simulink model "SistemaP2"  (R2024b)
settings: Solver=ode15s  StartTime=0.0  StopTime=30  RelTol=1e-3
libraries: slpidlib x1
settings Model: LastModifiedBy=DELL
settings DataIOCC: ReturnWorkspaceOutputs=off  TimeSaveName=t
settings DebuggingCC: AlgebraicLoopMsg=none  ArtificialAlgebraicLoopMsg=none  MaxConsecutiveZCsMsg=none  OperatingPointInterfaceChecksumMismatchMsg=none

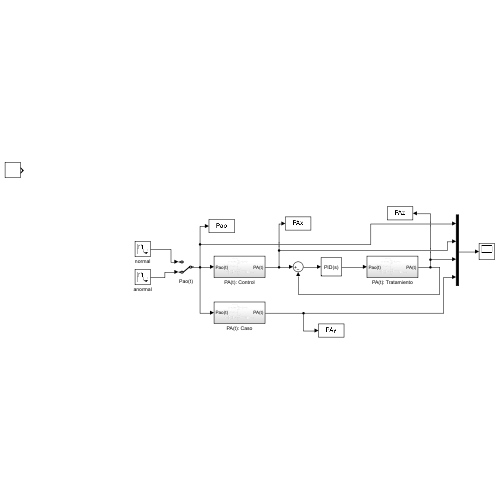
[thumbnail: Simulink's stored preview of the top-level diagram]
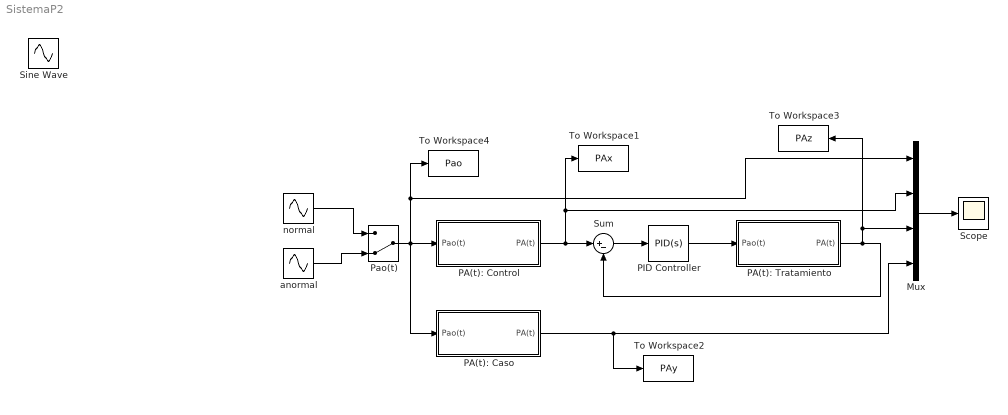
== system SistemaP2 ==
  Mux : Mux
  PA(t): Caso : Subsystem
  PA(t): Control : Subsystem
  PA(t): Tratamiento : Subsystem
  PID Controller : slpidlib/PID Controller  Controller=PID  Form=Parallel  TimeDomain=Continuous-time  UseExternalTs=off  SampleTime=-1  IntegratorMethod=Forward Euler  FilterMethod=Forward Euler  ControllerParametersSource=internal  P=151.384729406451  I=3438.58437249698  UseKiTs=off  D=0.496015778434629  UseExternalDerivativeSource=off  N=288.831749377284  UseFilter=on  TunerSelectOption=Transfer Function Based (PID Tuner App)  InitialConditionSource=internal  InitialConditionForIntegrator=0  InitialConditionForFilter=0  DifferentiatorICPrevScaledInput=0  ExternalReset=none  TrackingMode=off  Kt=1  LimitOutput=off  SatLimitsSource=internal  UpperSaturationLimit=inf  LowerSaturationLimit=-inf  LinearizeAsGain=on  AntiWindupMode=none  Kb=1  LimitIntegrator=off  UpperIntegratorSaturationLimit=inf  LowerIntegratorSaturationLimit=-inf  POutMin=[]  POutMax=[]  IOutMin=[]  IOutMax=[]  DOutMin=[]  DOutMax=[]  NOutMin=[]  NOutMax=[]  SumOutMin=[]  SumOutMax=[]  SaturationOutMin=[]  SaturationOutMax=[]  PParamMin=[]  PParamMax=[]  IParamMin=[]  IParamMax=[]  DParamMin=[]  DParamMax=[]  NParamMin=[]  NParamMax=[]  KbParamMin=[]  KbParamMax=[]  KtParamMin=[]  KtParamMax=[]  KbOutMin=[]  KbOutMax=[]  KtOutMin=[]  KtOutMax=[]  IntegratorOutMin=[]  IntegratorOutMax=[]  FilterOutMin=[]  FilterOutMax=[]  SumI1OutMin=[]  SumI1OutMax=[]  SumI2OutMin=[]  SumI2OutMax=[]  SumI3OutMin=[]  SumI3OutMax=[]  SumI4OutMin=[]  SumI4OutMax=[]  SumDOutMin=[]  SumDOutMax=[]  DifferentiatorOutMin=[]  DifferentiatorOutMax=[]  FilterDiffOutCoefMin=[]  FilterDiffOutCoefMax=[]  ReciprocalOutMin=[]  ReciprocalOutMax=[]  SumDenOutMin=[]  SumDenOutMax=[]  SumNumOutMin=[]  SumNumOutMax=[]  DivideOutMin=[]  DivideOutMax=[]  UdiffTsProdOutMin=[]  UdiffTsProdOutMax=[]  NTsProdOutMin=[]  NTsProdOutMax=[]  UintegralTsProdOutMin=[]  UintegralTsProdOutMax=[]  UngainTsProdOutMin=[]  UngainTsProdOutMax=[]  ClampingZeroOutDataTypeStr=Inherit: Inherit via back propagation  ClampingZeroOutMin=[]  ClampingZeroOutMax=[]  FilterDenConstantOutDataTypeStr=Inherit: Inherit via back propagation  FilterDenConstantOutMin=[]  FilterDenConstantOutMax=[]  PCopyOutDataTypeStr=Inherit: Inherit via back propagation  PCopyOutMin=[]  PCopyOutMax=[]  NCopyOutDataTypeStr=Inherit: Inherit via back propagation  NCopyOutMin=[]  NCopyOutMax=[]  IntegratorContinuousStateAttributes=''  IntegratorStateMustResolveToSignalObject=off  IntegratorRTWStateStorageClass=Auto  FilterContinuousStateAttributes=''  FilterStateMustResolveToSignalObject=off  FilterRTWStateStorageClass=Auto  ParallelPVariant=InternalParameters  IdealPVariant=Disabled  IVariant=InternalParameters  DVariant=InternalParameters  IntegratorVariant=Continuous  SatVariant=Disabled  AWVariant=Passthrough  PCopyVariant=Disabled  TRVariant=Disabled  FdbkBlocksVariant=Forward  IdealPFdbkVariant=Disabled  SatFdbkVariant=Disabled  DerivativeFilterVariant=ContFilter  NVariant=InternalParameters  NCopyVariant=Disabled  FilterICVariant=InternalICsFilter  IntegratorICVariant=InternalICs  ExternalResetVariant=Disabled  TRSumVariant=Passthrough  SumFdbkVariant=Disabled  SumVariant=Sum_PID  TsampFilterVariant=InternalTs  TsampNgainVariant=Passthrough  TsampIntegralVariant=Disabled_SignalSpec  ExternalSaturationOutDataTypeStr=Inherit: Same as second input  DerivativeSourceVariant=ErrorSignal  PreIntVariant=InternalPreInt
  Pao(t) : ManualSwitch  CurrentSetting=0
  Scope : Scope
  Sine Wave : Sin  Frequency=1.5708  SampleTime=0.001
  Sum : Sum  Inputs=|+-
  To Workspace1 : ToWorkspace  VariableName=PAx  SampleTime=-1
      settings: Save2DSignal=2-D array (concatenate along first dimension)
  To Workspace2 : ToWorkspace  VariableName=PAy  SampleTime=-1
      settings: Save2DSignal=2-D array (concatenate along first dimension)
  To Workspace3 : ToWorkspace  VariableName=PAz  SampleTime=-1
      settings: Save2DSignal=2-D array (concatenate along first dimension)
  To Workspace4 : ToWorkspace  VariableName=Pao  SampleTime=-1
      settings: Save2DSignal=2-D array (concatenate along first dimension)
  anormal : Sin  Amplitude=1.7  Frequency=pi  SampleTime=0.001
  normal : Sin  Amplitude=2.7  Frequency=pi/2  SampleTime=0.001
  wires:
  PA(t): Control/1(PA(t)) -> To Workspace1/1, Mux/2, Sum/1
  Sum/1 -> PID Controller/1
  Mux/1 -> Scope/1
  PA(t): Caso/1(PA(t)) -> To Workspace2/1, Mux/4
  PA(t): Tratamiento/1(PA(t)) -> Sum/2, To Workspace3/1, Mux/3
  PID Controller/1 -> PA(t): Tratamiento/1(Pao(t))
  Pao(t)/1 -> PA(t): Caso/1(Pao(t)), Mux/1, To Workspace4/1, PA(t): Control/1(Pao(t))
  anormal/1 -> Pao(t)/2
  normal/1 -> Pao(t)/1

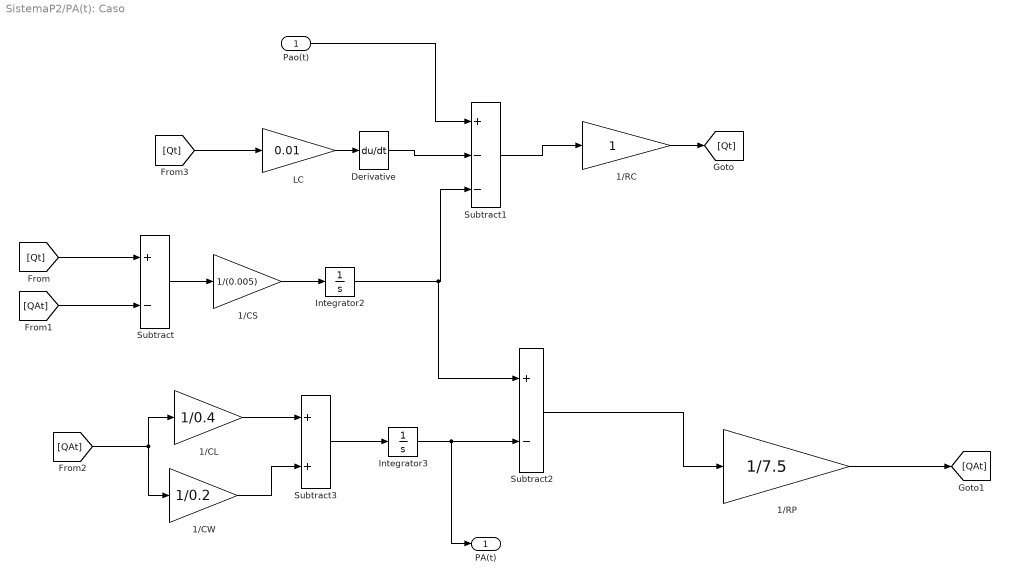
== system SistemaP2/PA(t): Caso ==
  Pao(t) : Inport
  1/CL : Gain  Gain=1/0.4
  1/CS : Gain  Gain=1/(0.005)
  1/CW : Gain  Gain=1/0.2
  1/RC : Gain
  1/RP : Gain  Gain=1/7.5
  Derivative : Derivative
  Integrator2 : Integrator
  Integrator3 : Integrator
  LC : Gain  Gain=0.01
  Subtract : Sum  Inputs=+-
  Subtract1 : Sum  Inputs=+--
  Subtract2 : Sum  Inputs=+-
  Subtract3 : Sum
  PA(t) : Outport
  wires:
  Pao(t)/1 -> Subtract1/1
  1/CS/1 -> Integrator2/1
  [Qt] -> Subtract/1
  LC/1 -> Derivative/1
  1/RC/1 -> [Qt]
  Subtract3/1 -> Integrator3/1
  [Qt] -> LC/1
  Integrator3/1 -> PA(t)/1, Subtract2/2
  1/CW/1 -> Subtract3/2
  Subtract1/1 -> 1/RC/1
  1/CL/1 -> Subtract3/1
  Subtract/1 -> 1/CS/1
  Integrator2/1 -> Subtract2/1, Subtract1/3
  Subtract2/1 -> 1/RP/1
  [QAt] -> Subtract/2
  1/RP/1 -> [QAt]
  Derivative/1 -> Subtract1/2
  [QAt] -> 1/CL/1, 1/CW/1

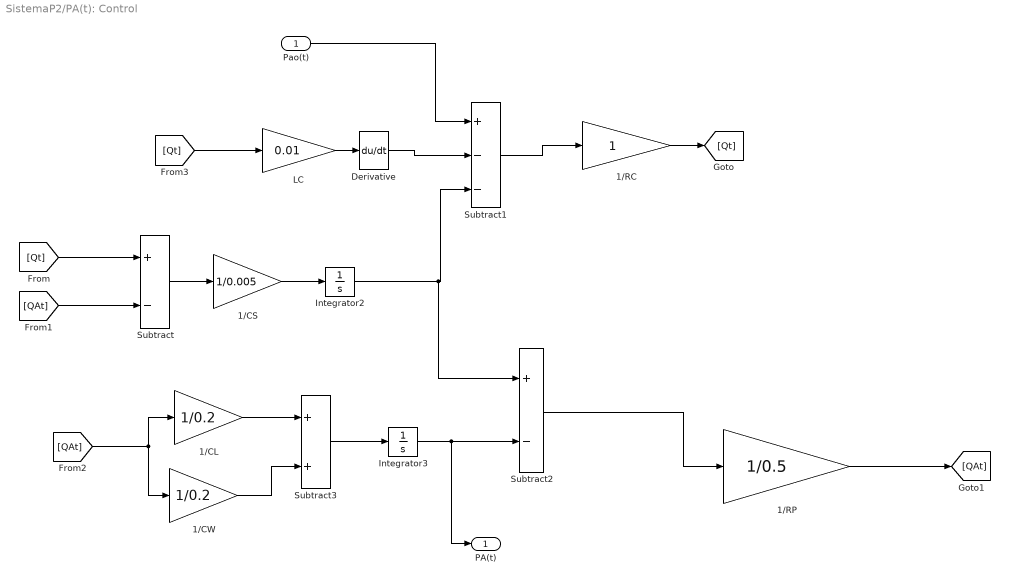
== system SistemaP2/PA(t): Control ==
  Pao(t) : Inport
  1/CL : Gain  Gain=1/0.2
  1/CS : Gain  Gain=1/0.005
  1/CW : Gain  Gain=1/0.2
  1/RC : Gain
  1/RP : Gain  Gain=1/0.5
  Derivative : Derivative
  Integrator2 : Integrator
  Integrator3 : Integrator
  LC : Gain  Gain=0.01
  Subtract : Sum  Inputs=+-
  Subtract1 : Sum  Inputs=+--
  Subtract2 : Sum  Inputs=+-
  Subtract3 : Sum
  PA(t) : Outport
  wires:
  1/RP/1 -> [QAt]
  Integrator2/1 -> Subtract2/1, Subtract1/3
  1/CS/1 -> Integrator2/1
  1/RC/1 -> [Qt]
  Subtract1/1 -> 1/RC/1
  Pao(t)/1 -> Subtract1/1
  Derivative/1 -> Subtract1/2
  LC/1 -> Derivative/1
  [QAt] -> Subtract/2
  [Qt] -> Subtract/1
  1/CW/1 -> Subtract3/2
  1/CL/1 -> Subtract3/1
  Subtract2/1 -> 1/RP/1
  [QAt] -> 1/CL/1, 1/CW/1
  [Qt] -> LC/1
  Subtract/1 -> 1/CS/1
  Subtract3/1 -> Integrator3/1
  Integrator3/1 -> PA(t)/1, Subtract2/2

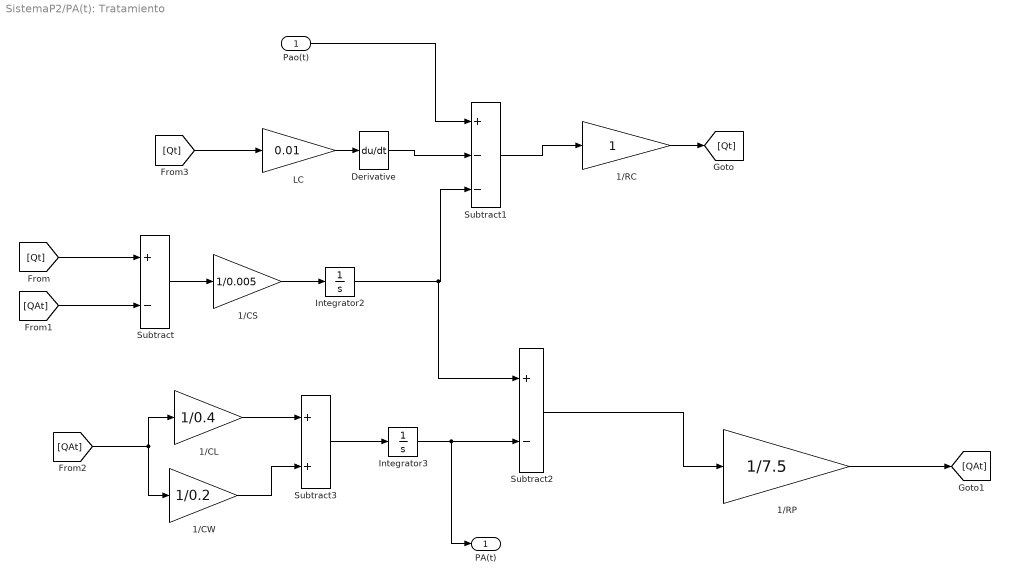
== system SistemaP2/PA(t): Tratamiento ==
  Pao(t) : Inport
  1/CL : Gain  Gain=1/0.4
  1/CS : Gain  Gain=1/0.005
  1/CW : Gain  Gain=1/0.2
  1/RC : Gain
  1/RP : Gain  Gain=1/7.5
  Derivative : Derivative
  Integrator2 : Integrator
  Integrator3 : Integrator
  LC : Gain  Gain=0.01
  Subtract : Sum  Inputs=+-
  Subtract1 : Sum  Inputs=+--
  Subtract2 : Sum  Inputs=+-
  Subtract3 : Sum
  PA(t) : Outport
  wires:
  Pao(t)/1 -> Subtract1/1
  1/CS/1 -> Integrator2/1
  [Qt] -> Subtract/1
  LC/1 -> Derivative/1
  1/RC/1 -> [Qt]
  Subtract3/1 -> Integrator3/1
  [Qt] -> LC/1
  Integrator3/1 -> PA(t)/1, Subtract2/2
  1/CW/1 -> Subtract3/2
  Subtract1/1 -> 1/RC/1
  1/CL/1 -> Subtract3/1
  Subtract/1 -> 1/CS/1
  Integrator2/1 -> Subtract2/1, Subtract1/3
  Subtract2/1 -> 1/RP/1
  [QAt] -> Subtract/2
  1/RP/1 -> [QAt]
  Derivative/1 -> Subtract1/2
  [QAt] -> 1/CL/1, 1/CW/1
